simulink model "Boiler_Demo"  (Simulink 6.0)
settings: Solver=ode23s  StartTime=0.0  StopTime=7200  RelTol=1e-5
model workspace (MAT data in the model file):
  SatSteam.Pressure = [0.8; 2; 5; 10; 20; 28; 35; 45; 55; 65; 75; 85; 95; 100; 101.33; 110; 130; 150; 170; 190; 220; 260; 280; 320; 360; 400; 440; 480; 500; 550; 600; 650; 700; 750; 800; 850; 900; 950; 1000; 1050; 1150; 1250; 1300; 1500; 1600; 1800; 2000; 2100; 2300; 2400; 2600; 2700; 2900; 3000; 3200; 3400; 3600; 3800; 4000]
  SatSteam.Temperature = [3.8; 17.5; 32.9; 45.8; 60.1; 67.5; 72.7; 78.7; 83.7; 88; 91.8; 95.2; 98.2; 99.6; 100; 102.3; 107.1; 111.4; 115.2; 118.6; 123.3; 128.7; 131.2; 135.8; 139.9; 143.1; 147.1; 150.3; 151.8; 155.5; 158.8; 162; 165; 167.8; 170.4; 172.9; 175.4; 177.7; 179.9; 182; 186; 189.8; 191.6; 198.3; 201.4; 207.1; 212.4; 214.9; 219.6; 221.8; 226; 228.1; 232; 233.8; 237.4; 240.9; 244.2; 247.3; 250.3]
  SatSteam.Volume = [160; 67; 28.2; 14.7; 7.65; 5.58; 4.53; 3.58; 2.96; 2.53; 2.22; 1.97; 1.78; 1.69; 1.67; 1.55; 1.33; 1.16; 1.03; 0.929; 0.81; 0.693; 0.646; 0.57; 0.51; 0.462; 0.423; 0.389; 0.375; 0.342; 0.315; 0.292; 0.273; 0.255; 0.24; 0.229; 0.215; 0.204; 0.194; 0.186; 0.17; 0.157; 0.151; 0.132; 0.124; 0.11; 0.0995; 0.0945; 0.0868; 0.0832; 0.0769; 0.074; 0.0689; 0.0666; 0.0624; 0.0587; 0.0554; 0.0524; 0.0497]
  SatSteam.Density = [0.00626; 0.0149; 0.0354; 0.0682; 0.131; 0.179; 0.221; 0.279; 0.338; 0.395; 0.45; 0.507; 0.563; 0.59; 0.598; 0.646; 0.755; 0.863; 0.97; 1.08; 1.23; 1.44; 1.55; 1.75; 1.96; 2.16; 2.36; 2.57; 2.67; 2.92; 3.175; 3.425; 3.66; 3.915; 4.16; 4.41; 4.65; 4.9; 5.15; 5.39; 5.89; 6.38; 6.62; 7.59; 8.03; 9.07; 10.01; 10.54; 11.52; 12.02; 13.01; 13.52; 14.52; 15; 16.02; 17.04; 18.06; 19.08; 21]
  SatSteam.EnthalpyLiquid = [15.8; 73.5; 137.8; 191.8; 251.5; 282.7; 304.3; 329.6; 350.6; 368.6; 384.5; 398.6; 411.5; 417.5; 419.1; 428.8; 449.2; 467.1; 483.2; 497.8; 517.6; 540.9; 551.4; 570.9; 588.5; 604.7; 619.6; 633.5; 640.1; 655.8; 670.4; 684.1; 697.1; 709.3; 720.9; 732; 742.6; 752.8; 762.6; 772; 790; 807; 815; 845; 859; 885; 909; 920; 942; 952; 972; 981; 1000; 1008; 1025; 1042; 1058; 1073; 1087]
  SatSteam.EnthalpyEvaporation = [2493; 2460; 2424; 2393; 2358; 2340; 2327; 2312; 2299; 2288; 2279; 2270; 2262; 2258; 2257; 2251; 2238; 2226; 2216; 2206; 2193; 2177; 2170; 2157; 2144; 2133; 2122; 2112; 2107; 2096; 2085; 2075; 2065; 2056; 2047; 2038; 2030; 2021; 2014; 2006; 1991; 1977; 1971; 1945; 1933; 1910; 1889; 1878; 1858; 1849; 1830; 1821; 1803; 1794; 1779; 1760; 1744; 1728; 1713]
  SatSteam.EnthalpySteam = [2509; 2534; 2562; 2585; 2610; 2623; 2632; 2642; 2650; 2657; 2663; 2668; 2673; 2675; 2676; 2680; 2687; 2698; 2699; 2704; 2711; 2718; 2722; 2728; 2733; 2738; 2742; 2746; 2748; 2752; 2756; 2759; 2762; 2765; 2768; 2770; 2772; 2774; 2776; 2778; 2781; 2784; 2785; 2790; 2792; 2795; 2797; 2798; 2800; 2800; 2801; 2802; 2802; 2802; 2802; 2802; 2802; 2801; 2800]
  SatSteam.dp = [1.2; 3; 5; 10; 8; 7; 10; 10; 10; 10; 10; 10; 5; 1.33; 8.67; 20; 20; 20; 20; 30; 40; 20; 40; 40; 40; 40; 40; 20; 50; 50; 50; 50; 50; 50; 50; 50; 50; 50; 50; 100; 100; 50; 200; 100; 200; 200; 100; 200; 100; 200; 100; 200; 100; 200; 200; 200; 200; 200]
  SatSteam.dT = [13.7; 15.4; 12.9; 14.3; 7.4; 5.2; 6; 5; 4.3; 3.8; 3.4; 3; 1.4; 0.4; 2.3; 4.8; 4.3; 3.8; 3.4; 4.7; 5.4; 2.5; 4.6; 4.1; 3.2; 4; 3.2; 1.5; 3.7; 3.3; 3.2; 3; 2.8; 2.6; 2.5; 2.5; 2.3; 2.2; 2.1; 4; 3.8; 1.8; 6.7; 3.1; 5.7; 5.3; 2.5; 4.7; 2.2; 4.2; 2.1; 3.9; 1.8; 3.6; 3.5; 3.3; 3.1; 3]
  SatSteam.drho_by_dp = [0.0072; 0.00683333333333; 0.00656; 0.00628; 0.006; 0.006; 0.0058; 0.0059; 0.0057; 0.0055; 0.0057; 0.0056; 0.0054; 0.00601503759398; 0.00553633217993; 0.00545; 0.0054; 0.00535; 0.0055; 0.005; 0.00525; 0.0055; 0.005; 0.00525; 0.005; 0.005; 0.00525; 0.005; 0.005; 0.0051; 0.005; 0.0047; 0.0051; 0.0049; 0.005; 0.0048; 0.005; 0.005; 0.0048; 0.005; 0.0049; 0.0048; 0.00485; 0.0044; 0.0052; 0.0047; 0.0053; 0.0049; 0.005; 0.00495; 0.0051; 0.005; 0.0048; 0.0051; 0.0051; 0.0051; 0.0051; 0.0096]
  SatSteam.dhw_by_dp = [48.0833333333; 21.4333333333; 10.8; 5.97; 3.9; 3.08571428571; 2.53; 2.1; 1.8; 1.59; 1.41; 1.29; 1.2; 1.2030075188; 1.11880046136; 1.02; 0.895; 0.805; 0.73; 0.66; 0.5825; 0.525; 0.4875; 0.44; 0.405; 0.3725; 0.3475; 0.33; 0.314; 0.292; 0.274; 0.26; 0.244; 0.232; 0.222; 0.212; 0.204; 0.196; 0.188; 0.18; 0.17; 0.16; 0.15; 0.14; 0.13; 0.12; 0.11; 0.11; 0.1; 0.1; 0.09; 0.095; 0.08; 0.085; 0.085; 0.08; 0.075; 0.07]
  SatSteam.dhs_by_dp = [20.8333333333; 9.33333333333; 4.6; 2.5; 1.625; 1.28571428571; 1; 0.8; 0.7; 0.6; 0.5; 0.5; 0.4; 0.751879699248; 0.461361014994; 0.35; 0.55; 0.05; 0.25; 0.233333333333; 0.175; 0.2; 0.15; 0.125; 0.125; 0.1; 0.1; 0.1; 0.08; 0.08; 0.06; 0.06; 0.06; 0.06; 0.04; 0.04; 0.04; 0.04; 0.04; 0.03; 0.03; 0.02; 0.025; 0.02; 0.015; 0.01; 0.01; 0.01; 0; 0.005; 0.01; 0; 0; 0; 0; 0; -0.005; -0.005]
  SatSteam.dt_by_dp = [11.4166666667; 5.13333333333; 2.58; 1.43; 0.925; 0.742857142857; 0.6; 0.5; 0.43; 0.38; 0.34; 0.3; 0.28; 0.300751879699; 0.265282583622; 0.24; 0.215; 0.19; 0.17; 0.156666666667; 0.135; 0.125; 0.115; 0.1025; 0.08; 0.1; 0.08; 0.075; 0.074; 0.066; 0.064; 0.06; 0.056; 0.052; 0.05; 0.05; 0.046; 0.044; 0.042; 0.04; 0.038; 0.036; 0.0335; 0.031; 0.0285; 0.0265; 0.025; 0.0235; 0.022; 0.021; 0.021; 0.0195; 0.018; 0.018; 0.0175; 0.0165; 0.0155; 0.015]
  SatSteam.drho_by_dT = [0.000630656934307; 0.00133116883117; 0.00254263565891; 0.00439160839161; 0.00648648648649; 0.00807692307692; 0.00966666666667; 0.0118; 0.0132558139535; 0.0144736842105; 0.0167647058824; 0.0186666666667; 0.0192857142857; 0.02; 0.0208695652174; 0.0227083333333; 0.0251162790698; 0.0281578947368; 0.0323529411765; 0.031914893617; 0.0388888888889; 0.044; 0.0434782608696; 0.0512195121951; 0.0625; 0.05; 0.065625; 0.0666666666667; 0.0675675675676; 0.0772727272727; 0.078125; 0.0783333333333; 0.0910714285714; 0.0942307692308; 0.1; 0.096; 0.108695652174; 0.113636363636; 0.114285714286; 0.125; 0.128947368421; 0.133333333333; 0.144776119403; 0.141935483871; 0.182456140351; 0.177358490566; 0.212; 0.208510638298; 0.227272727273; 0.235714285714; 0.242857142857; 0.25641025641; 0.266666666667; 0.283333333333; 0.291428571429; 0.309090909091; 0.329032258065; 0.64]
  SatSteam.dhw_by_dT = [4.21167883212; 4.17532467532; 4.18604651163; 4.17482517483; 4.21621621622; 4.15384615385; 4.21666666667; 4.2; 4.18604651163; 4.18421052632; 4.14705882353; 4.3; 4.28571428571; 4; 4.21739130435; 4.25; 4.16279069767; 4.23684210526; 4.29411764706; 4.21276595745; 4.31481481481; 4.2; 4.23913043478; 4.29268292683; 5.0625; 3.725; 4.34375; 4.4; 4.24324324324; 4.42424242424; 4.28125; 4.33333333333; 4.35714285714; 4.46153846154; 4.44; 4.24; 4.4347826087; 4.45454545455; 4.47619047619; 4.5; 4.47368421053; 4.44444444444; 4.4776119403; 4.51612903226; 4.56140350877; 4.52830188679; 4.4; 4.68085106383; 4.54545454545; 4.7619047619; 4.28571428571; 4.87179487179; 4.44444444444; 4.72222222222; 4.85714285714; 4.84848484848; 4.83870967742; 4.66666666667]
  SatSteam.dhs_by_dT = [1.82481751825; 1.81818181818; 1.78294573643; 1.74825174825; 1.75675675676; 1.73076923077; 1.66666666667; 1.6; 1.62790697674; 1.57894736842; 1.47058823529; 1.66666666667; 1.42857142857; 2.5; 1.73913043478; 1.45833333333; 2.55813953488; 0.263157894737; 1.47058823529; 1.48936170213; 1.2962962963; 1.6; 1.30434782609; 1.21951219512; 1.5625; 1; 1.25; 1.33333333333; 1.08108108108; 1.21212121212; 0.9375; 1; 1.07142857143; 1.15384615385; 0.8; 0.8; 0.869565217391; 0.909090909091; 0.952380952381; 0.75; 0.789473684211; 0.555555555556; 0.746268656716; 0.645161290323; 0.526315789474; 0.377358490566; 0.4; 0.425531914894; 0; 0.238095238095; 0.47619047619; 0; 0; 0; 0; 0; -0.322580645161; -0.333333333333]
  SatSteam.dp_by_dT = [0.0875912408759; 0.194805194805; 0.387596899225; 0.699300699301; 1.08108108108; 1.34615384615; 1.66666666667; 2; 2.32558139535; 2.63157894737; 2.94117647059; 3.33333333333; 3.57142857143; 3.325; 3.76956521739; 4.16666666667; 4.6511627907; 5.26315789474; 5.88235294118; 6.3829787234; 7.40740740741; 8; 8.69565217391; 9.75609756098; 12.5; 10; 12.5; 13.3333333333; 13.5135135135; 15.1515151515; 15.625; 16.6666666667; 17.8571428571; 19.2307692308; 20; 20; 21.7391304348; 22.7272727273; 23.8095238095; 25; 26.3157894737; 27.7777777778; 29.8507462687; 32.2580645161; 35.0877192982; 37.7358490566; 40; 42.5531914894; 45.4545454545; 47.619047619; 47.619047619; 51.2820512821; 55.5555555556; 55.5555555556; 57.1428571429; 60.6060606061; 64.5161290323; 66.6666666667]
  Tw = 88
  Mt = 20000
  Cp = 452
  Vt = 8
  Pout = 101
  Kfout = 3.3352
  HeatDistAmplitude = 40000
  rhoWater = 1000
  T0 = 180
  Tmin : num (value not decoded)
PreLoadFcn:
  | u0 = zeros(2,1);
  | y0 = zeros(1,1);
  | K = tf( {0;0}, 1);
  | Kobsv = ss(eye(2),zeros(2,3),zeros(2,2),zeros(2,3));
libraries: cstblocks x2
settings Model: Creator=astother  LastModifiedBy=jglass  BufferReuse=off
settings DataIOCC: SignalLoggingName=logsOut
settings OptimizationCC: InlineParams=on  BufferReuse=off
settings DebuggingCC: CheckExecutionContextPreStartOutputMsg=on  CheckExecutionContextRuntimeOutputMsg=on  SolverPrmCheckMsg=none

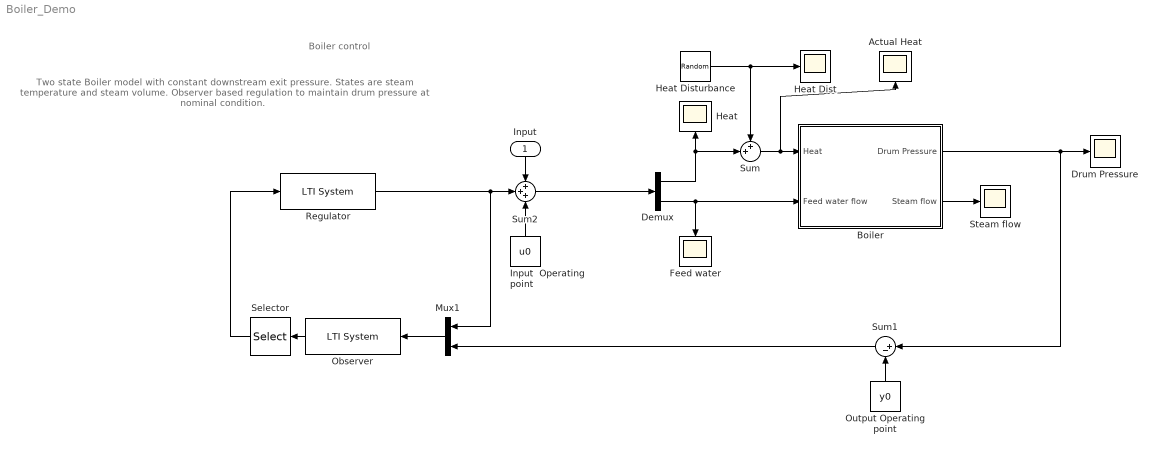
== system Boiler_Demo ==
  note: Two state Boiler model with constant downstream exit pressure.
      | States are steam temperature and steam volume. Observer based regulation
      | to maintain drum pressure at nominal condition.
  note: Boiler control
  Input : Inport  Orientation=down  PortDimensions=2  LatchInput=off
  Actual Heat : Scope
      settings: Orientation=up  TimeRange=4000  YMin=240200  YMax=240800  SaveName=ActualHeat
  Boiler : Subsystem  PropExecContextAcrossSSBoundary=on
  Demux : Demux  Outputs=2
  Drum Pressure : Scope
      settings: TimeRange=8000  YMin=990  YMax=1015  SaveName=DrumPressure
  Feed water : Scope
      settings: Orientation=down  TimeRange=8000  YMin=92  YMax=106  SaveName=FeedWater
  Heat : Scope
      settings: Orientation=up  TimeRange=8000  YMin=240950  YMax=241200  SaveName=Heat
  Heat Dist : Scope
      settings: TimeRange=4000  YMin=-150000  YMax=200000  SaveName=HeatDist
  Heat Disturbance : RandomNumber  Variance=HeatDistAmplitude^2  SampleTime=0
  Input  Operating point : Constant  Orientation=up  Value=u0
  Mux1 : Mux  Orientation=left  Inputs=2
  Observer : cstblocks/LTI System  Orientation=left  sys=Kobsv  IC=0
  Output Operating point : Constant  Orientation=up  Value=y0
  Regulator : cstblocks/LTI System  sys=-K  IC=[]
  Selector : Selector  Orientation=left  Elements=[2]  InputPortWidth=2
  Steam flow : Scope
      settings: TimeRange=4000  YMin=99.9  YMax=100.4
  Sum : Sum  Inputs=++|
  Sum1 : Sum  Orientation=left  Inputs=|+-
  Sum2 : Sum  Inputs=+++
  wires:
  Observer/1 -> Selector/1
  Boiler/2(Steam flow) -> Steam flow/1
  Boiler/1(Drum Pressure) -> Drum Pressure/1, Sum1/1
  Sum/1 -> Boiler/1(Heat), Actual Heat/1
  Demux/1 -> Sum/2, Heat/1
  Demux/2 -> Boiler/2(Feed water flow), Feed water/1
  Output Operating point/1 -> Sum1/2
  Mux1/1 -> Observer/1
  Sum1/1 -> Mux1/2
  Selector/1 -> Regulator/1
  Regulator/1 -> Mux1/1, Sum2/2
  Sum2/1 -> Demux/1
  Heat Disturbance/1 -> Heat Dist/1, Sum/1
  Input  Operating point/1 -> Sum2/3
  Input/1 -> Sum2/1

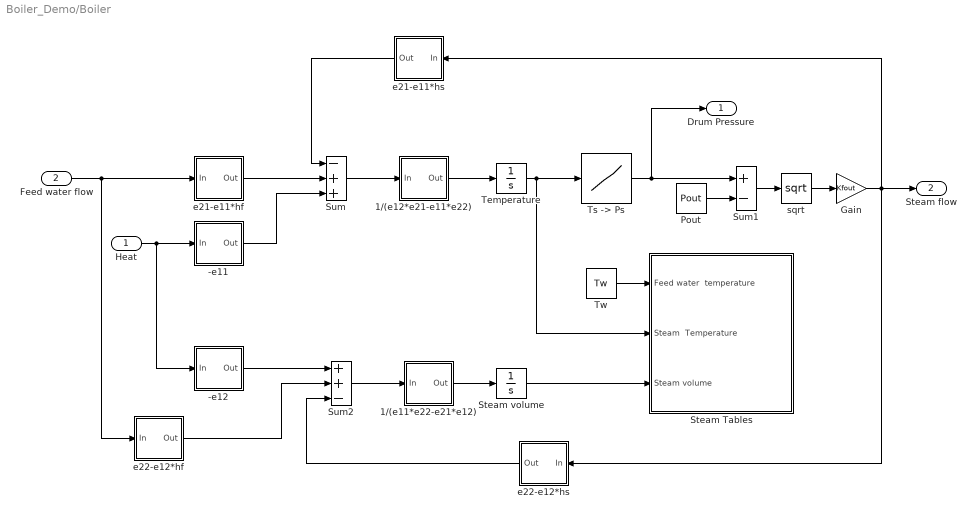
== system Boiler_Demo/Boiler ==
  Heat : Inport  PortDimensions=1  LatchInput=off
  Feed water flow : Inport  Port=2  PortDimensions=1  LatchInput=off
  -e11 : Subsystem  PropExecContextAcrossSSBoundary=on
  -e12 : Subsystem  PropExecContextAcrossSSBoundary=on
  1/(e11*e22-e21*e12) : Subsystem  PropExecContextAcrossSSBoundary=on
  1/(e12*e21-e11*e22) : Subsystem  PropExecContextAcrossSSBoundary=on
  Gain : Gain  Gain=Kfout
  Pout : Constant  Value=Pout
  Steam Tables : Subsystem  PropExecContextAcrossSSBoundary=on
  Steam volume : Integrator  InitialCondition=0.7*Vt  LimitOutput=on  LowerSaturationLimit=0
  Sum : Sum  Inputs=-++
  Sum1 : Sum  Inputs=+-
  Sum2 : Sum  Inputs=++-
  Temperature : Integrator  InitialCondition=T0  LimitOutput=on  LowerSaturationLimit=Tmin
  "Ts -> Ps" : Lookup  DialogController=Simulink.DDGSource  InputValues=SatSteam.Temperature  OutputValues=SatSteam.Pressure
  Tw : Constant  Value=Tw
  e21-e11*hf : Subsystem  PropExecContextAcrossSSBoundary=on
  e21-e11*hs : Subsystem  Orientation=left  PropExecContextAcrossSSBoundary=on
  e22-e12*hf : Subsystem  PropExecContextAcrossSSBoundary=on
  e22-e12*hs : Subsystem  Orientation=left  PropExecContextAcrossSSBoundary=on
  sqrt : Math  Operator=sqrt  SaturateOnIntegerOverflow=on
  Drum Pressure : Outport  PortDimensions=1
  Steam flow : Outport  Port=2  PortDimensions=1
  wires:
  1/(e12*e21-e11*e22)/1(Out) -> Temperature/1
  Sum/1 -> 1/(e12*e21-e11*e22)/1(In)
  Heat/1 -> -e11/1(In), -e12/1(In)
  -e11/1(Out) -> Sum/3
  e21-e11*hf/1(Out) -> Sum/2
  Feed water flow/1 -> e21-e11*hf/1(In), e22-e12*hf/1(In)
  e21-e11*hs/1(Out) -> Sum/1
  1/(e11*e22-e21*e12)/1(Out) -> Steam volume/1
  Sum2/1 -> 1/(e11*e22-e21*e12)/1(In)
  e22-e12*hs/1(Out) -> Sum2/3
  -e12/1(Out) -> Sum2/1
  e22-e12*hf/1(Out) -> Sum2/2
  Tw/1 -> Steam Tables/1(Feed water  temperature)
  Temperature/1 -> Steam Tables/2(Steam  Temperature), "Ts -> Ps"/1
  Pout/1 -> Sum1/2
  Sum1/1 -> sqrt/1
  sqrt/1 -> Gain/1
  Gain/1 -> Steam flow/1, e21-e11*hs/1(In), e22-e12*hs/1(In)
  Steam volume/1 -> Steam Tables/3(Steam volume)
  "Ts -> Ps"/1 -> Sum1/1, Drum Pressure/1

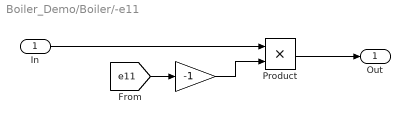
== system Boiler_Demo/Boiler/-e11 ==
  In : Inport  LatchInput=off
  " " : Gain  Gain=-1
  Product : Product  RndMeth=Zero
  Out : Outport
  wires:
  In/1 -> Product/1
  Product/1 -> Out/1
  [e11] -> " "/1
  " "/1 -> Product/2

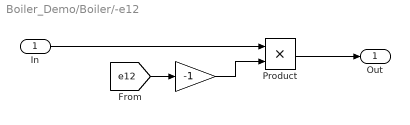
== system Boiler_Demo/Boiler/-e12 ==
  In : Inport  LatchInput=off
  " " : Gain  Gain=-1
  Product : Product  RndMeth=Zero
  Out : Outport
  wires:
  In/1 -> Product/1
  Product/1 -> Out/1
  [e12] -> " "/1
  " "/1 -> Product/2

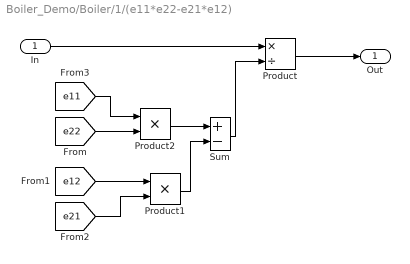
== system Boiler_Demo/Boiler/1/(e11*e22-e21*e12) ==
  In : Inport  LatchInput=off
  Product : Product  Inputs=*/  RndMeth=Zero
  Product1 : Product  RndMeth=Zero
  Product2 : Product  RndMeth=Zero
  Sum : Sum  Inputs=+-
  Out : Outport
  wires:
  In/1 -> Product/1
  Product/1 -> Out/1
  [e12] -> Product1/1
  [e21] -> Product1/2
  Product1/1 -> Sum/2
  Sum/1 -> Product/2
  Product2/1 -> Sum/1
  [e22] -> Product2/2
  [e11] -> Product2/1

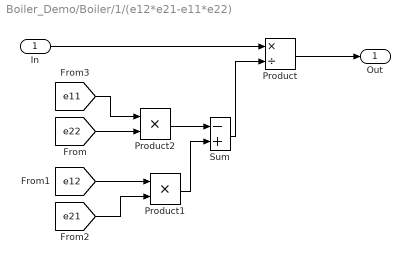
== system Boiler_Demo/Boiler/1/(e12*e21-e11*e22) ==
  In : Inport  LatchInput=off
  Product : Product  Inputs=*/  RndMeth=Zero
  Product1 : Product  RndMeth=Zero
  Product2 : Product  RndMeth=Zero
  Sum : Sum  Inputs=-+
  Out : Outport
  wires:
  In/1 -> Product/1
  Product/1 -> Out/1
  [e12] -> Product1/1
  [e21] -> Product1/2
  Product1/1 -> Sum/2
  Sum/1 -> Product/2
  Product2/1 -> Sum/1
  [e22] -> Product2/2
  [e11] -> Product2/1

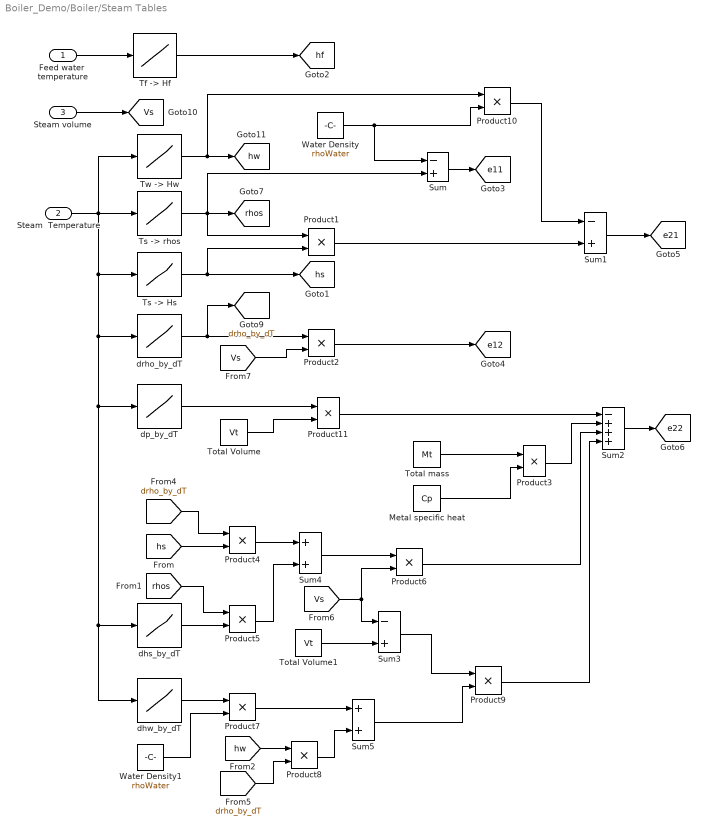
== system Boiler_Demo/Boiler/Steam Tables ==
  Feed water  temperature : Inport  LatchInput=off
  Steam  Temperature : Inport  Port=2  LatchInput=off
  Steam volume : Inport  Port=3  LatchInput=off
  Metal specific heat : Constant  Value=Cp
  Product{1..11} (11 alike) : Product  RndMeth=Zero
  Sum : Sum  Inputs=-+
  Sum1 : Sum  Inputs=-+
  Sum2 : Sum  Inputs=-+++
  Sum3 : Sum  Inputs=-+
  Sum4 : Sum
  Sum5 : Sum
  "Tf -> Hf" : Lookup  DialogController=Simulink.DDGSource  InputValues=SatSteam.Temperature  OutputValues=SatSteam.EnthalpyLiquid
  Total Volume : Constant  Value=Vt
  Total Volume1 : Constant  Value=Vt
  Total mass : Constant  Value=Mt
  "Ts -> Hs" : Lookup  DialogController=Simulink.DDGSource  InputValues=SatSteam.Temperature  OutputValues=SatSteam.EnthalpySteam
  "Ts -> rhos" : Lookup  DialogController=Simulink.DDGSource  InputValues=SatSteam.Temperature  OutputValues=SatSteam.Density
  "Tw -> Hw" : Lookup  DialogController=Simulink.DDGSource  InputValues=SatSteam.Temperature  OutputValues=SatSteam.EnthalpyLiquid
  Water Density : Constant  Value=rhoWater
  Water Density1 : Constant  Value=rhoWater
  dhs_by_dT : Lookup  DialogController=Simulink.DDGSource  InputValues=SatSteam.Temperature(2:end)  OutputValues=SatSteam.dhs_by_dT
  dhw_by_dT : Lookup  DialogController=Simulink.DDGSource  InputValues=SatSteam.Temperature(2:end)  OutputValues=SatSteam.dhw_by_dp
  dp_by_dT : Lookup  DialogController=Simulink.DDGSource  InputValues=SatSteam.Temperature(2:end)  OutputValues=SatSteam.dp_by_dT
  drho_by_dT : Lookup  DialogController=Simulink.DDGSource  InputValues=SatSteam.Temperature(2:end)  OutputValues=SatSteam.drho_by_dT
  tag scope: Vs=global, drho_by_dT=global, e11=global, e12=global, e21=global, e22=global, hf=global, hs=global, hw=global, rhos=global
  wires:
  "Ts -> Hs"/1 -> [hs], Product1/2
  "Tf -> Hf"/1 -> [hf]
  Feed water  temperature/1 -> "Tf -> Hf"/1
  Sum/1 -> [e11]
  Water Density/1 -> Sum/1, Product10/2
  Steam  Temperature/1 -> "Ts -> rhos"/1, "Ts -> Hs"/1, drho_by_dT/1, dp_by_dT/1, dhs_by_dT/1, dhw_by_dT/1, "Tw -> Hw"/1
  "Ts -> rhos"/1 -> Sum/2, Product1/1, [rhos]
  Sum1/1 -> [e21]
  Product1/1 -> Sum1/2
  drho_by_dT/1 -> Product2/1, [drho_by_dT]
  Product2/1 -> [e12]
  Sum2/1 -> [e22]
  Metal specific heat/1 -> Product3/2
  Product3/1 -> Sum2/2
  [hs] -> Product4/2
  dhs_by_dT/1 -> Product5/2
  [rhos] -> Product5/1
  Product4/1 -> Sum4/1
  Product5/1 -> Sum4/2
  Sum4/1 -> Product6/1
  Product6/1 -> Sum2/3
  dhw_by_dT/1 -> Product7/1
  [hw] -> Product8/1
  [drho_by_dT] -> Product4/1
  [drho_by_dT] -> Product8/2
  Product8/1 -> Sum5/2
  Product7/1 -> Sum5/1
  Sum5/1 -> Product9/2
  Product9/1 -> Sum2/4
  [Vs] -> Product2/2
  "Tw -> Hw"/1 -> Product10/1, [hw]
  Product10/1 -> Sum1/1
  [Vs] -> Product6/2, Sum3/1
  Total Volume1/1 -> Sum3/2
  Sum3/1 -> Product9/1
  Steam volume/1 -> [Vs]
  Total mass/1 -> Product3/1
  dp_by_dT/1 -> Product11/1
  Total Volume/1 -> Product11/2
  Product11/1 -> Sum2/1
  Water Density1/1 -> Product7/2

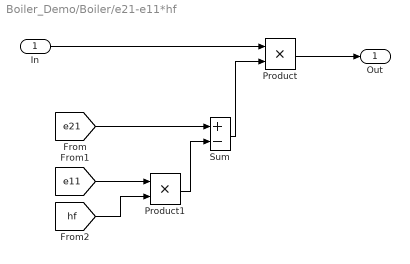
== system Boiler_Demo/Boiler/e21-e11*hf ==
  In : Inport  LatchInput=off
  Product : Product  RndMeth=Zero
  Product1 : Product  RndMeth=Zero
  Sum : Sum  Inputs=+-
  Out : Outport
  wires:
  In/1 -> Product/1
  Product/1 -> Out/1
  [e11] -> Product1/1
  [hf] -> Product1/2
  Product1/1 -> Sum/2
  Sum/1 -> Product/2
  [e21] -> Sum/1

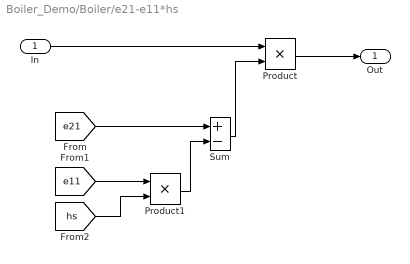
== system Boiler_Demo/Boiler/e21-e11*hs ==
  In : Inport  LatchInput=off
  Product : Product  RndMeth=Zero
  Product1 : Product  RndMeth=Zero
  Sum : Sum  Inputs=+-
  Out : Outport
  wires:
  In/1 -> Product/1
  Product/1 -> Out/1
  [e11] -> Product1/1
  [hs] -> Product1/2
  Product1/1 -> Sum/2
  Sum/1 -> Product/2
  [e21] -> Sum/1

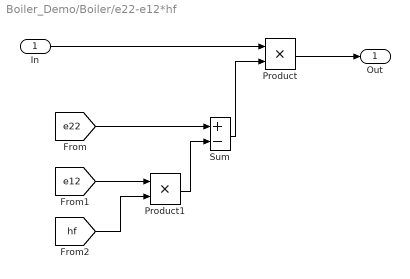
== system Boiler_Demo/Boiler/e22-e12*hf ==
  In : Inport  LatchInput=off
  Product : Product  RndMeth=Zero
  Product1 : Product  RndMeth=Zero
  Sum : Sum  Inputs=+-
  Out : Outport
  wires:
  In/1 -> Product/1
  Product/1 -> Out/1
  [e12] -> Product1/1
  [hf] -> Product1/2
  [e22] -> Sum/1
  Product1/1 -> Sum/2
  Sum/1 -> Product/2

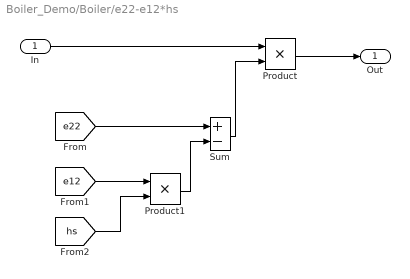
== system Boiler_Demo/Boiler/e22-e12*hs ==
  In : Inport  LatchInput=off
  Product : Product  RndMeth=Zero
  Product1 : Product  RndMeth=Zero
  Sum : Sum  Inputs=+-
  Out : Outport
  wires:
  In/1 -> Product/1
  Product/1 -> Out/1
  [e12] -> Product1/1
  [hs] -> Product1/2
  [e22] -> Sum/1
  Product1/1 -> Sum/2
  Sum/1 -> Product/2
